simulink model "Lap2"  (R2021a)
settings: Solver=FixedStepAuto  StartTime=0.0  StopTime=10.0  FixedStep=1e-3  RelTol=1e-3
settings Model: Creator=lenovo  LastModifiedBy=lenovo

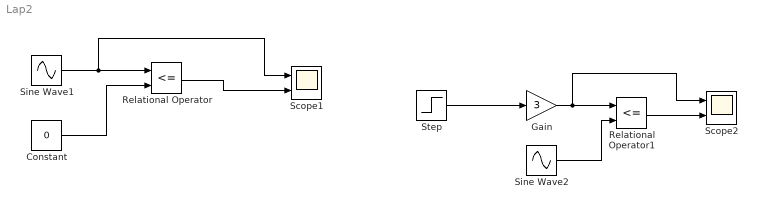
== system Lap2 ==
  Constant : Constant  Value=0
  Gain : Gain  Gain=3
  Relational Operator : RelationalOperator  Operator=<=  OutDataTypeStr=boolean  RndMeth=Simplest
  Relational Operator1 : RelationalOperator  Operator=<=  OutDataTypeStr=boolean  RndMeth=Simplest
  Scope1 : Scope  NumInputPorts=2
  Scope2 : Scope  NumInputPorts=2
  Sine Wave1 : Sin  Frequency=2*pi*1  SampleTime=0
  Sine Wave2 : Sin  Frequency=2*pi*1  SampleTime=0
  Step : Step  Time=2  SampleTime=0
  wires:
  Sine Wave1/1 -> Scope1/1, Relational Operator/1
  Constant/1 -> Relational Operator/2
  Relational Operator/1 -> Scope1/2
  Step/1 -> Gain/1
  Relational Operator1/1 -> Scope2/2
  Gain/1 -> Scope2/1, Relational Operator1/1
  Sine Wave2/1 -> Relational Operator1/2
